simulink model "Ramp1"  (R2024b)
settings: Solver=VariableStepAuto  StartTime=0.0  StopTime=10.0  RelTol=1e-3
libraries: simulink x3
settings Model: Creator=Ahmad  LastModifiedBy=Ahmad

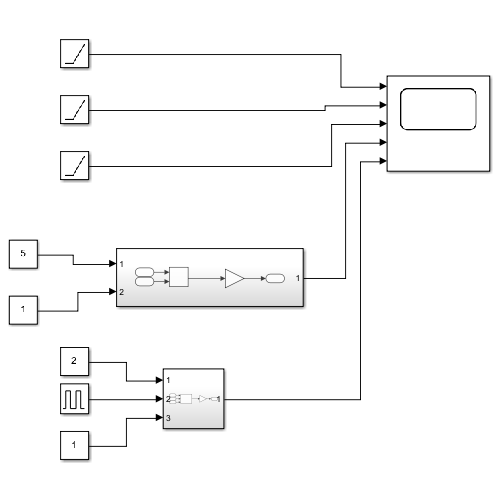
[thumbnail: Simulink's stored preview of the top-level diagram]
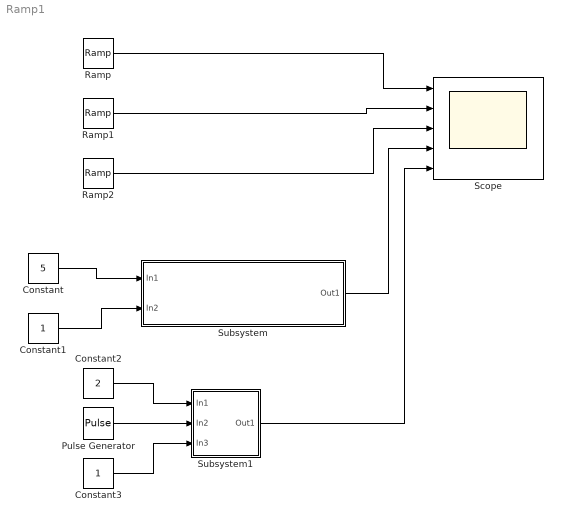
== system Ramp1 ==
  Constant : Constant  Value=5
  Constant1 : Constant
  Constant2 : Constant  Value=2
  Constant3 : Constant
  Pulse Generator : DiscretePulseGenerator  PulseType=Time based  Period=10  PulseWidth=50
  Ramp : simulink/Sources/Ramp  slope=5  start=3  InitialOutput=0
  Ramp1 : simulink/Sources/Ramp  slope=-5  start=2  InitialOutput=0
  Ramp2 : simulink/Sources/Ramp  slope=1  start=0  InitialOutput=4
  Scope : Scope  NumInputPorts=5
  Subsystem : Subsystem
  Subsystem1 : Subsystem
  wires:
  Ramp/1 -> Scope/1
  Ramp1/1 -> Scope/2
  Ramp2/1 -> Scope/3
  Constant/1 -> Subsystem/1(In1)
  Constant1/1 -> Subsystem/2(In2)
  Subsystem/1(Out1) -> Scope/4
  Constant2/1 -> Subsystem1/1(In1)
  Pulse Generator/1 -> Subsystem1/2(In2)
  Constant3/1 -> Subsystem1/3(In3)
  Subsystem1/1(Out1) -> Scope/5

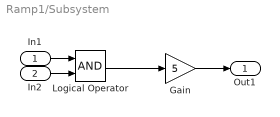
== system Ramp1/Subsystem ==
  In1 : Inport
  In2 : Inport  Port=2
  Gain : Gain  Gain=5
  Logical Operator : Logic  AllPortsSameDT=off  OutDataTypeStr=boolean
  Out1 : Outport
  wires:
  Gain/1 -> Out1/1
  In1/1 -> Logical Operator/1
  In2/1 -> Logical Operator/2
  Logical Operator/1 -> Gain/1

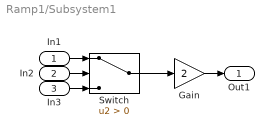
== system Ramp1/Subsystem1 ==
  In1 : Inport
  In2 : Inport  Port=2
  In3 : Inport  Port=3
  Gain : Gain  Gain=2
  Switch : Switch  Criteria=u2 > Threshold  SaturateOnIntegerOverflow=off  InputSameDT=off
  Out1 : Outport
  wires:
  In1/1 -> Switch/1
  Switch/1 -> Gain/1
  In3/1 -> Switch/3
  In2/1 -> Switch/2
  Gain/1 -> Out1/1
